simulink model "comsat_model"  (R2015b)
settings: Solver=FixedStepAuto  SolverMode=SingleTasking  StartTime=t_s  StopTime=t_e  FixedStep=dt  RelTol=1e-3
values from neighbouring files (symbols this model uses):
  A = [ ... (first row only)    [comsat_data.m]
  B = [ ... (first row only)    [comsat_data.m]
  C = eye(3,3)    [comsat_data.m]
  D = zeros(3,1)    [comsat_data.m]
  dt = 0.1    [main.m]
  init = [0 0 0.0587]    [main.m]
settings Model: Creator=yakov  LastModifiedBy=79534
settings DataIOCC: LimitDataPoints=off  ReturnWorkspaceOutputs=on
settings OptimizationCC: DefaultParameterBehavior=Inlined  OptimizeModelRefInitCode=on
settings DebuggingCC: AllowSymbolicDim=on  SFUnexpectedBacktrackingDiag=error  SFNoUnconditionalDefaultTransitionDiag=error
settings HardwareCC: TargetBitPerPointer=64  TargetLongLongMode=on  TargetIntDivRoundTo=Zero  TargetEndianess=LittleEndian  TargetWordSize=64  TargetHWDeviceType=MATLAB Host  ProdEqTarget=off
settings ModelReferenceCC: PropagateSignalLabelsOutOfModel=on
settings SFSimCC: SimUseLocalCustomCode=on
settings RTWCC: Description=Embedded Coder (host-based shared library target)  SystemTargetFile=ert_shrlib.tlc  GenCodeOnly=on  TemplateMakefile=ert_default_tmf  RTWUseLocalCustomCode=on
settings CodeAppCC: IgnoreCustomStorageClasses=off
settings STFCustomTargetCC: GenerateSampleERTMain=on  ParMdlRefBuildCompliant=on  CompOptLevelCompliant=on  ConcurrentExecutionCompliant=off  GeneratePreprocessorConditionals=Use local settings  CombineOutputUpdateFcns=on  ERTCustomFileBanners=on  SupportNonInlinedSFcns=off  MATLABClassNameForMDSCustomization=Simulink.SoftwareTarget.ERTCustomization  ModelStepFunctionPrototypeControlCompliant=on  CPPClassGenCompliant=off  GRTInterface=off  UseToolchainInfoCompliant=on  SystemTargetFile=ert_shrlib.tlc
settings ERTTargetCC: GenerateSampleERTMain=on  ConcurrentExecutionCompliant=off  SupportContinuousTime=on  CPPClassGenCompliant=off  InlinedParameterPlacement=NonHierarchical  ERTCustomFileTemplate=example_file_process.tlc
settings ConfigComp: CovMetricSettings=dwe  CovSaveCumulativeToWorkspaceVar=off  CovSaveSingleToWorkspaceVar=off  CovModelRefEnable=Off  CovExternalEMLEnable=on

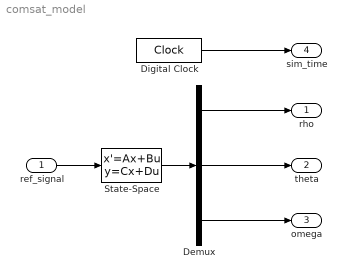
== system comsat_model ==
  ref_signal : Inport
  Demux : Demux  Outputs=3
  Digital Clock : DigitalClock  SampleTime=dt
  State-Space : StateSpace  A=A  B=B  C=C  D=D  X0=init
  rho : Outport
  theta : Outport  Port=2
  omega : Outport  Port=3
  "sim_time " : Outport  Port=4
  wires:
  ref_signal/1 -> State-Space/1
  Demux/2 -> theta/1
  State-Space/1 -> Demux/1
  Demux/1 -> rho/1
  Demux/3 -> omega/1
  Digital Clock/1 -> "sim_time "/1
